simulink model "collison"  (R2020a)
settings: Solver=VariableStepAuto  StartTime=0.0  StopTime=10.0  RelTol=1e-3
settings Model: Creator=Mayukh  LastModifiedBy=sarka

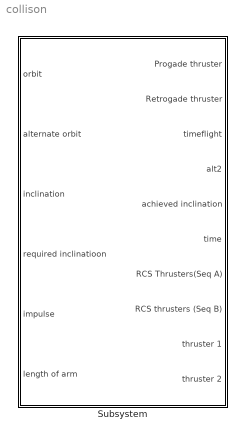
== system collison ==
  Subsystem : Subsystem

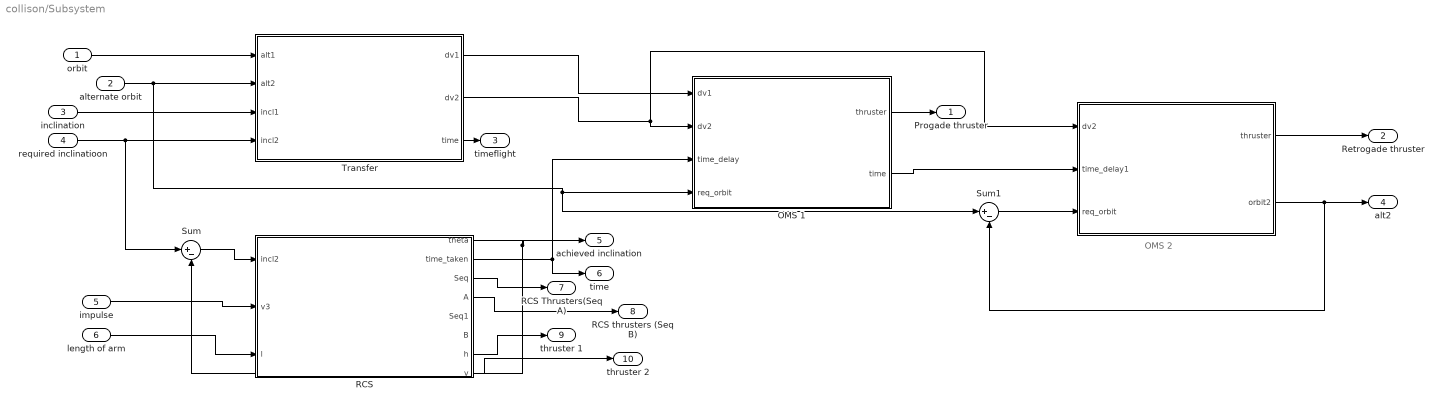
== system collison/Subsystem ==
  note: OMS 2
  orbit : Inport
  alternate orbit : Inport  Port=2
  inclination : Inport  Port=3
  required inclinatioon : Inport  Port=4
  impulse : Inport  Port=5
  length of arm : Inport  Port=6
  " " : MATLAB Function  TreatAsAtomicUnit=on
  OMS 1 : MATLAB Function  TreatAsAtomicUnit=on
  RCS : MATLAB Function  TreatAsAtomicUnit=on
  Sum : Sum  Inputs=|+-
  Sum1 : Sum  Inputs=|+-
  Transfer : MATLAB Function  TreatAsAtomicUnit=on
  "Progade thruster " : Outport
  Retrogade thruster : Outport  Port=2
  timeflight : Outport  Port=3
  "alt2 " : Outport  Port=4
  achieved inclination : Outport  Port=5
  time : Outport  Port=6
  RCS Thrusters(Seq A) : Outport  Port=7
  RCS thrusters (Seq B) : Outport  Port=8
  "thruster 1 " : Outport  Port=9
  "thruster 2 " : Outport  Port=10
  wires:
  required inclinatioon/1 -> Sum/1, Transfer/4(incl2)
  impulse/1 -> RCS/2(v3)
  alternate orbit/1 -> Sum1/1, OMS 1/4(req_orbit), Transfer/2(alt2)
  Sum/1 -> RCS/1(incl2)
  inclination/1 -> Transfer/3(incl1)
  Transfer/2(dv2) -> " "/1(dv2), OMS 1/2(dv2)
  RCS/1(theta) -> achieved inclination/1, Sum/2
  Transfer/1(dv1) -> OMS 1/1(dv1)
  " "/2(orbit2) -> "alt2 "/1, Sum1/2
  RCS/2(time_taken) -> time/1, OMS 1/3(time_delay)
  Sum1/1 -> " "/3(req_orbit)
  RCS/4(A) -> RCS thrusters (Seq B)/1
  OMS 1/1(thruster) -> "Progade thruster "/1
  length of arm/1 -> RCS/3(l)
  " "/1(thruster) -> Retrogade thruster/1
  RCS/3(Seq) -> RCS Thrusters(Seq A)/1
  RCS/7(h) -> "thruster 1 "/1
  orbit/1 -> Transfer/1(alt1)
  RCS/8(v) -> "thruster 2 "/1
  Transfer/3(time) -> timeflight/1
  OMS 1/2(time) -> " "/2(time_delay1)

== matlab function collison/Subsystem/RCS ==
  data: incl2 input; theta output; v3 input; l input; time_taken output; Seq output; A output; Seq1 output; B output; h output; v output
function [theta,time_taken , Seq,A , Seq1,B,h ,v] = fcn(incl2 , v3 , l)

y = u;

== matlab function collison/Subsystem/Transfer ==
  data: alt1 input; dv1 output; alt2 input; incl1 input; incl2 input; dv2 output; time output
function [dv1 , dv2 , time] = fcn(alt1 , alt2 , incl1 ,incl2)

y = u;

== matlab function collison/Subsystem/OMS 1 ==
  data: dv1 input; thruster output; dv2 input; time_delay input; req_orbit input; time output
function [thruster , time] = fcn(dv1 , dv2 , time_delay, req_orbit)

y = u;

== matlab function collison/Subsystem/  ==
  data: dv2 input; time_delay1 input; thruster output; req_orbit input; orbit2 output
function [thruster , orbit2] = fcn(  dv2 , time_delay1, req_orbit)

y = u;
